simulink model "FBmodel"  (R2022b)
settings: Solver=VariableStepAuto  StartTime=0.0  StopTime=5  MaxStep=0.01  RelTol=1e-3
values from neighbouring files (symbols this model uses):
  dot_x_des = length/t_des    [DataEstimationAndConstraints.m]
  friction = friction(:,1:numSample)    [DataReading.m]    (also in DataSampling.m = random(frictionUniformDist, 1, numSample); SensitivityAnalysisConfig.m = 0.5; data.mat = [0.423870600502 0.414714985315 0.508364191084 0.585845302695)
  g = random(gDist, 1, 1)    [DataSampling.m]    (also in SensitivityAnalysisConfig.m = 9.8; data.mat = 9.78798650818)
  PID = [3, 0.5, 0]    [DataEstimationAndConstraints.m]
  weight = weight(:,1:numSample)    [DataReading.m]    (also in DataSampling.m = random(weightDist, 1, numSample); SensitivityAnalysisConfig.m = 0.025; data.mat = [0.0249399431455 0.0249880813357 0.0249204436802 0.024988815)
libraries: simulink x1, slpidlib x1
settings Model: Creator=w.ar  LastModifiedBy=w.ar

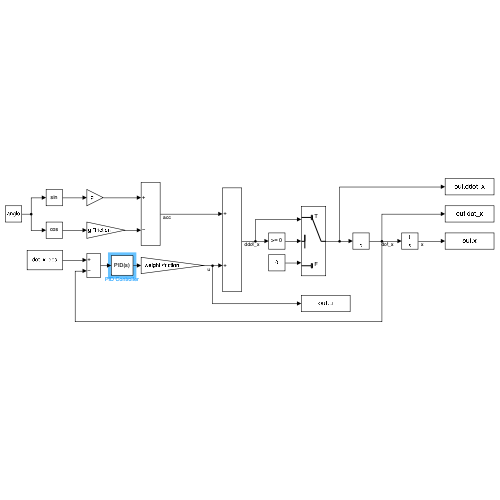
[thumbnail: Simulink's stored preview of the top-level diagram]
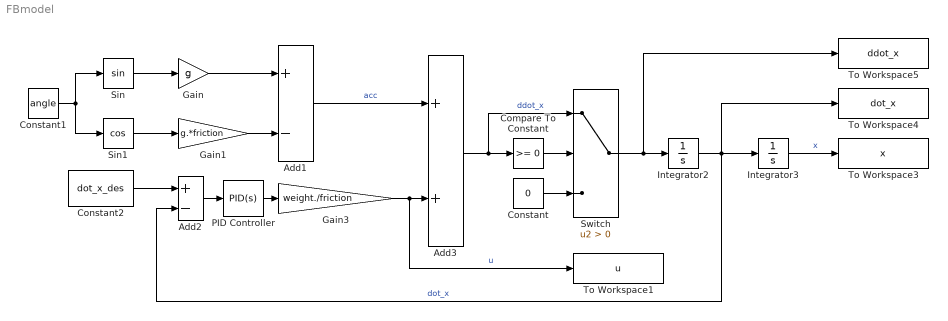
== system FBmodel ==
  Add1 : Sum  Inputs=+-
  Add2 : Sum  Inputs=+-
  Add3 : Sum
  Compare To Constant : simulink/Logic and Bit Operations/Compare To Constant  relop=>=  const=0  OutDataTypeStr=boolean
  Constant : Constant  Value=0
  Constant1 : Constant  Value=angle
  Constant2 : Constant  Value=dot_x_des
  Gain : Gain  Gain=g
  Gain1 : Gain  Gain=g.*friction
  Gain3 : Gain  Gain=weight./friction
  Integrator2 : Integrator
  Integrator3 : Integrator  UpperSaturationLimit=length
  PID Controller : slpidlib/PID Controller  Controller=PID  Form=Parallel  TimeDomain=Continuous-time  UseExternalTs=off  SampleTime=-1  IntegratorMethod=Forward Euler  FilterMethod=Forward Euler  ControllerParametersSource=internal  P=PID(1)  I=PID(2)  UseKiTs=off  D=PID(3)  N=100  UseFilter=on  TunerSelectOption=Transfer Function Based (PID Tuner App)  InitialConditionSource=internal  InitialConditionForIntegrator=0  InitialConditionForFilter=0  DifferentiatorICPrevScaledInput=0  ExternalReset=none  TrackingMode=off  Kt=1  LimitOutput=off  SatLimitsSource=internal  UpperSaturationLimit=inf  LowerSaturationLimit=-inf  LinearizeAsGain=on  AntiWindupMode=none  Kb=1  LimitIntegrator=off  UpperIntegratorSaturationLimit=inf  LowerIntegratorSaturationLimit=-inf  POutMin=[]  POutMax=[]  IOutMin=[]  IOutMax=[]  DOutMin=[]  DOutMax=[]  NOutMin=[]  NOutMax=[]  SumOutMin=[]  SumOutMax=[]  SaturationOutMin=[]  SaturationOutMax=[]  PParamMin=[]  PParamMax=[]  IParamMin=[]  IParamMax=[]  DParamMin=[]  DParamMax=[]  NParamMin=[]  NParamMax=[]  KbParamMin=[]  KbParamMax=[]  KtParamMin=[]  KtParamMax=[]  KbOutMin=[]  KbOutMax=[]  KtOutMin=[]  KtOutMax=[]  IntegratorOutMin=[]  IntegratorOutMax=[]  FilterOutMin=[]  FilterOutMax=[]  SumI1OutMin=[]  SumI1OutMax=[]  SumI2OutMin=[]  SumI2OutMax=[]  SumI3OutMin=[]  SumI3OutMax=[]  SumI4OutMin=[]  SumI4OutMax=[]  SumDOutMin=[]  SumDOutMax=[]  DifferentiatorOutMin=[]  DifferentiatorOutMax=[]  FilterDiffOutCoefMin=[]  FilterDiffOutCoefMax=[]  ReciprocalOutMin=[]  ReciprocalOutMax=[]  SumDenOutMin=[]  SumDenOutMax=[]  SumNumOutMin=[]  SumNumOutMax=[]  DivideOutMin=[]  DivideOutMax=[]  UdiffTsProdOutMin=[]  UdiffTsProdOutMax=[]  NTsProdOutMin=[]  NTsProdOutMax=[]  UintegralTsProdOutMin=[]  UintegralTsProdOutMax=[]  UngainTsProdOutMin=[]  UngainTsProdOutMax=[]  ClampingZeroOutDataTypeStr=Inherit: Inherit via back propagation  ClampingZeroOutMin=[]  ClampingZeroOutMax=[]  FilterDenConstantOutDataTypeStr=Inherit: Inherit via back propagation  FilterDenConstantOutMin=[]  FilterDenConstantOutMax=[]  PCopyOutDataTypeStr=Inherit: Inherit via back propagation  PCopyOutMin=[]  PCopyOutMax=[]  NCopyOutDataTypeStr=Inherit: Inherit via back propagation  NCopyOutMin=[]  NCopyOutMax=[]  IntegratorContinuousStateAttributes=''  IntegratorStateMustResolveToSignalObject=off  IntegratorRTWStateStorageClass=Auto  FilterContinuousStateAttributes=''  FilterStateMustResolveToSignalObject=off  FilterRTWStateStorageClass=Auto  ParallelPVariant=InternalParameters  IdealPVariant=Disabled  IVariant=InternalParameters  DVariant=InternalParameters  IntegratorVariant=Continuous  SatVariant=Disabled  AWVariant=Passthrough  PCopyVariant=Disabled  TRVariant=Disabled  FdbkBlocksVariant=Forward  IdealPFdbkVariant=Disabled  SatFdbkVariant=Disabled  DerivativeFilterVariant=ContFilter  NVariant=InternalParameters  NCopyVariant=Disabled  FilterICVariant=InternalICsFilter  IntegratorICVariant=InternalICs  ExternalResetVariant=Disabled  TRSumVariant=Passthrough  SumFdbkVariant=Disabled  SumVariant=Sum_PID  TsampFilterVariant=InternalTs  TsampNgainVariant=Passthrough  TsampIntegralVariant=Passthrough  ExternalSaturationOutDataTypeStr=Inherit: Same as second input
  Sin : Trigonometry
  Sin1 : Trigonometry  Operator=cos
  Switch : Switch  Criteria=u2 > Threshold  SaturateOnIntegerOverflow=off  InputSameDT=off
  To Workspace1 : ToWorkspace  VariableName=u  SaveFormat=Timeseries  SampleTime=-1
  To Workspace3 : ToWorkspace  VariableName=x  SaveFormat=Timeseries  SampleTime=-1
  To Workspace4 : ToWorkspace  VariableName=dot_x  SaveFormat=Timeseries  SampleTime=-1
  To Workspace5 : ToWorkspace  VariableName=ddot_x  SaveFormat=Timeseries  SampleTime=-1
  wires:
  Constant1/1 -> Sin1/1, Sin/1
  Sin1/1 -> Gain1/1
  Sin/1 -> Gain/1
  Gain/1 -> Add1/1
  Gain1/1 -> Add1/2
  Constant2/1 -> Add2/1
  Add1/1 -> Add3/1  "acc"
  Gain3/1 -> To Workspace1/1, Add3/2  "u"
  Integrator2/1 -> Add2/2, To Workspace4/1, Integrator3/1  "dot_x"
  Integrator3/1 -> To Workspace3/1  "x"
  Add2/1 -> PID Controller/1
  PID Controller/1 -> Gain3/1
  Compare To Constant/1 -> Switch/2
  Add3/1 -> Switch/1, Compare To Constant/1  "ddot_x"
  Switch/1 -> To Workspace5/1, Integrator2/1
  Constant/1 -> Switch/3
